simulink model "CubeSat_ADCS_Nadir"  (R2024b)
settings: Solver=ode4  StartTime=0.0  StopTime=5000  FixedStep=T_sample  RelTol=1e-3
values from neighbouring files (symbols this model uses):
  B_mag = 40e-6    (= 4e-05)    [init_sim.m]
  Init_Quat = [1; 0; 0; 0]    [init_sim.m]
  Init_Rates = [0.0; -n_orbit; 0.0]    [init_sim.m]
  Init_Wheel_Speed = [0; 0; 0]    [init_sim.m]
  J_body = diag([0.002, 0.002, 0.002])    [init_sim.m]
  J_inv = inv(J_body)    [init_sim.m]
  J_wheel = diag([J_w_val, J_w_val, J_w_val])    [init_sim.m]
  J_wheel_inv = inv(J_wheel)    [init_sim.m]
  K_desat = 1e4    (= 10000)    [init_sim.m]
  Kd = 8e-3    (= 0.008)    [init_sim.m]
  Kp = 5e-4    (= 0.0005)    [init_sim.m]
  Max_Dipole = 0.2    [init_sim.m]
  n_orbit = 0.0011    [init_sim.m]
  Tau_Max = 1e-3    (= 0.001)    [init_sim.m]
settings Model: Creator=abdel  LastModifiedBy=abdel

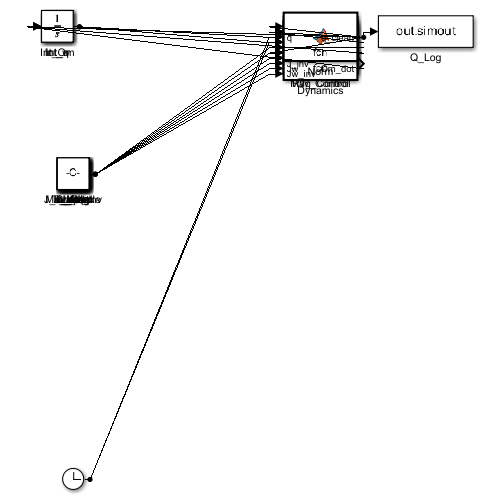
[thumbnail: Simulink's stored preview of the top-level diagram]
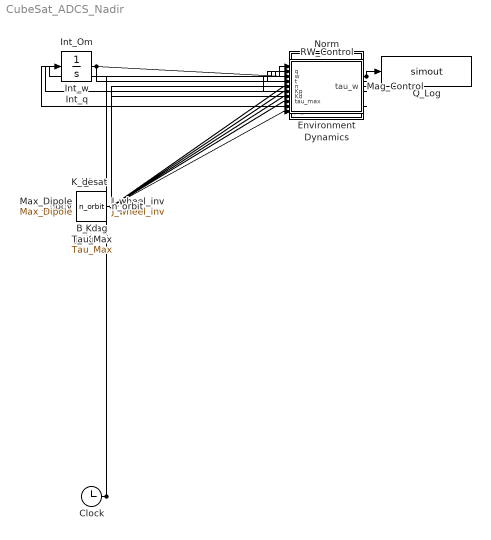
== system CubeSat_ADCS_Nadir ==
  B_mag : Constant  Value=B_mag
  Clock : Clock
  Dynamics : MATLAB Function  TreatAsAtomicUnit=on
  Environment : MATLAB Function  TreatAsAtomicUnit=on
  Int_Om : Integrator  InitialCondition=Init_Wheel_Speed
  Int_q : Integrator  InitialCondition=Init_Quat
  Int_w : Integrator  InitialCondition=Init_Rates
  J_body : Constant  Value=J_body
  J_inv : Constant  Value=J_inv
  J_wheel : Constant  Value=J_wheel
  J_wheel_inv : Constant  Value=J_wheel_inv
  K_desat : Constant  Value=K_desat
  Kd : Constant  Value=Kd
  Kp : Constant  Value=Kp
  Mag_Control : MATLAB Function  TreatAsAtomicUnit=on
  Max_Dipole : Constant  Value=Max_Dipole
  Norm : MATLAB Function  TreatAsAtomicUnit=on
  Q_Log : ToWorkspace  VariableName=simout  SampleTime=-1
  RW_Control : MATLAB Function  TreatAsAtomicUnit=on
  Tau_Max : Constant  Value=Tau_Max
  n_orbit : Constant  Value=n_orbit
  wires:
  Int_q/1 -> Norm/1(q)
  Norm/1(q_clean) -> Environment/1(q), RW_Control/1(q), Dynamics/1(q), Q_Log/1
  Clock/1 -> Environment/2(t), RW_Control/3(t)
  B_mag/1 -> Environment/3(B_mag)
  n_orbit/1 -> Environment/4(n), RW_Control/4(n)
  Int_w/1 -> RW_Control/2(w), Mag_Control/2(w), Dynamics/2(w)
  Kp/1 -> RW_Control/5(Kp)
  Kd/1 -> RW_Control/6(Kd)
  Tau_Max/1 -> RW_Control/7(tau_max)
  Environment/1(B_body) -> Mag_Control/1(B_body)
  Int_Om/1 -> Mag_Control/3(Om), Dynamics/3(Om)
  J_body/1 -> Mag_Control/4(J), Dynamics/6(J)
  J_wheel/1 -> Mag_Control/5(Jw), Dynamics/8(Jw)
  K_desat/1 -> Mag_Control/6(K)
  Max_Dipole/1 -> Mag_Control/7(m_max)
  RW_Control/1(tau_w) -> Dynamics/4(tau_w)
  Mag_Control/1(tau_mag) -> Dynamics/5(tau_mag)
  J_inv/1 -> Dynamics/7(J_inv)
  J_wheel_inv/1 -> Dynamics/9(Jw_inv)
  Dynamics/1(q_dot) -> Int_q/1
  Dynamics/2(w_dot) -> Int_w/1
  Dynamics/3(Om_dot) -> Int_Om/1

== matlab function CubeSat_ADCS_Nadir/Mag_Control ==
  data: B_body input; tau_mag output; w input; Om input; J input; Jw input; K input; m_max input; m_cmd output
function [tau_mag, m_cmd] = fcn(B_body, w, Om, J, Jw, K, m_max)
    H_total = J*w + Jw*Om;
    m_ideal = -K * cross(H_total, B_body);
    m_cmd = zeros(3,1);
    for i=1:3, m_cmd(i) = max(min(m_ideal(i), m_max), -m_max); end
    tau_mag = cross(m_cmd, B_body);
end

== matlab function CubeSat_ADCS_Nadir/Environment ==
  data: q input; B_body output; t input; B_mag input; n input
function B_body = fcn(q, t, B_mag, n)
    % Simple Rotating Magnetic Field Model
    B_inertial = B_mag * [cos(n*t); sin(n*t); 0.5*sin(2*n*t)];
    
    q_conj = [q(1); -q(2); -q(3); -q(4)];
    dcm = [1-2*(q(3)^2+q(4)^2), 2*(q(2)*q(3)+q(1)*q(4)), 2*(q(2)*q(4)-q(1)*q(3));
           2*(q(2)*q(3)-q(1)*q(4)), 1-2*(q(2)^2+q(4)^2), 2*(q(3)*q(4)+q(1)*q(2));
           2*(q(2)*q(4)+q(1)*q(3)), 2*(q(3)*q(4)-q(1)*q(2)), 1-2*(q(2)^2+q(3)^2)];
    B_body = dcm * B_inertial;
end

== matlab function CubeSat_ADCS_Nadir/RW_Control ==
  data: q input; tau_w output; w input; t input; n input; Kp input; Kd input; tau_max input
function tau_w = fcn(q, w, t, n, Kp, Kd, tau_max)
    tau_w = zeros(3,1);
    q = q(:); w = w(:);
    
    % 1. GENERATE MOVING TARGET (NADIR)
    % To point at Earth, we must pitch at rate 'n'
    % Angle theta = n * t
    theta = n * t;
    
    % Target Quaternion: Rotation about Y-axis by theta
    % (This assumes Y-axis is perpendicular to orbit plane)
    qt = [cos(theta/2); 0; sin(theta/2); 0];
    
    % 2. CALCULATE ERROR QUATERNION
    % q_err = q_target_conjugate * q_current
    qt_c = [qt(1); -qt(2); -qt(3); -qt(4)];
    
    % Quaternion Multiplication
    qe = zeros(4,1);
    qe(1) = qt_c(1)*q(1) - qt_c(2)*q(2) - qt_c(3)*q(3) - qt_c(4)*q(4);
    qe(2) = qt_c(1)*q(2) + qt_c(2)*q(1) + qt_c(3)*q(4) - qt_c(4)*q(3);
    qe(3) = qt_c(1)*q(3) - qt_c(2)*q(4) + qt_c(3)*q(1) + qt_c(4)*q(2);
    qe(4) = qt_c(1)*q(4) + qt_c(2)*q(3) - qt_c(3)*q(2) + qt_c(4)*q(1);
    
    % Shortest path check
    if qe(1) < 0, qe = -qe; end
    
    % 3. TARGET ANGULAR VELOCITY
    % We don't want to stop (w=0), we want to pitch (w = [0; n; 0])
    w_targ = [0; n; 0];
    w_err = w - w_targ;
    
    % 4. PD CONTROL
    e_vec = qe(2:4);
    tau_body_cmd = -Kp * e_vec - Kd * w_err;
    
    tau_w_raw = -tau_body_cmd;
    for i=1:3, tau_w(i) = max(min(tau_w_raw(i), tau_max), -tau_max); end
end

== matlab function CubeSat_ADCS_Nadir/Dynamics ==
  data: q input; q_dot output; w input; Om input; tau_w input; tau_mag input; J input; J_inv input; Jw input; Jw_inv input; w_dot output; Om_dot output
function [q_dot, w_dot, Om_dot] = fcn(q, w, Om, tau_w, tau_mag, J, J_inv, Jw, Jw_inv)
    q = q(:); w = w(:); Om = Om(:); tau_w = tau_w(:); tau_mag = tau_mag(:);
    q_dot = 0.5 * [ -q(2)*w(1) - q(3)*w(2) - q(4)*w(3);
                     q(1)*w(1) - q(4)*w(2) + q(3)*w(3);
                     q(4)*w(1) + q(1)*w(2) - q(2)*w(3);
                    -q(3)*w(1) + q(2)*w(2) + q(1)*w(3) ];
    H = J*w + Jw*Om;
    w_dot = J_inv * ( -tau_w + tau_mag - cross(w, H) );
    Om_dot = Jw_inv * tau_w;
end

== matlab function CubeSat_ADCS_Nadir/Norm ==
  data: q input; q_clean output
function q_clean = fcn(q)
    q = q(:); n = norm(q); if n < 1e-12, n = 1; end; q_clean = q / n;
end
